simulink model "pcssp_Voiture"  (R2021b)
settings: configuration reference "configurationSettings" (kept outside this file)
undefined symbols (not defined in the file or in its folder): pcssp_Voiture_tp
settings Model: DataDictionary=pcssp_Voiture.sldd  Creator=timoravensbergen  LastModifiedBy=timoravensbergen
settings ConfigSetRef: SourceName=configurationSettings

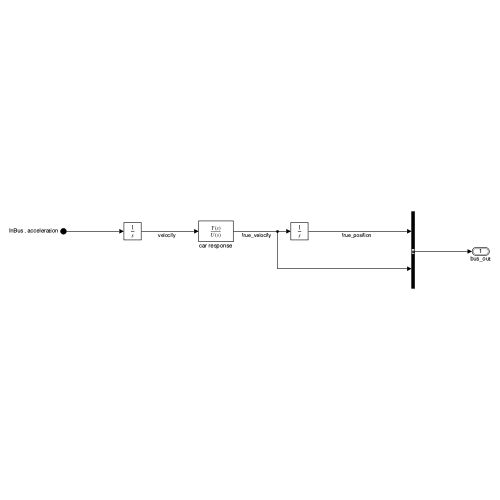
[thumbnail: Simulink's stored preview of the top-level diagram]
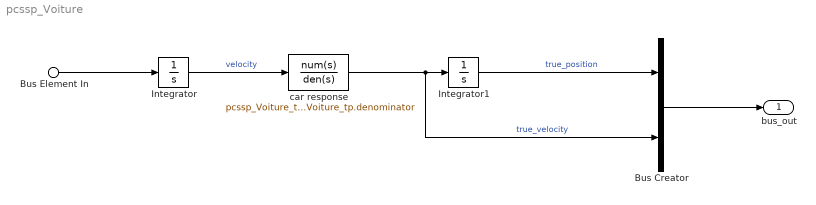
== system pcssp_Voiture ==
  Bus Element In : Inport  PortName=InBus  Element=acceleration
  Bus Creator : BusCreator  Inputs=2  OutDataTypeStr=Bus: pcssp_Voiture_outBus
      settings: InheritFromInputs=off
  Integrator : Integrator  InitialCondition=pcssp_Voiture_tp.v0
  Integrator1 : Integrator  InitialCondition=pcssp_Voiture_tp.s0
  car response : TransferFcn  Numerator=pcssp_Voiture_tp.numerator  Denominator=pcssp_Voiture_tp.denominator
  bus_out : Outport  OutDataTypeStr=Bus: pcssp_Voiture_outBus
  wires:
  Integrator/1 -> car response/1  "velocity"
  car response/1 -> Bus Creator/2, Integrator1/1  "true_velocity"
  Integrator1/1 -> Bus Creator/1  "true_position"
  Bus Creator/1 -> bus_out/1
  Bus Element In/1 -> Integrator/1
